simulink model "ExampleMotive_control_communication"  (R2016a)
settings: Solver=ode1  StartTime=0.0  StopTime=inf  FixedStep=0.2  RelTol=1e-3
settings Model: ExtModeTrigDuration=5000  Creator=adm-drone  LastModifiedBy=jitesh_esb201
settings SolverCC: PositivePriorityOrder=on
settings DataIOCC: LimitDataPoints=on  SaveFormat=Array
settings DebuggingCC: UnderspecifiedInitializationDetection=Classic  MergeDetectMultiDrivingBlocksExec=none  SolverPrmCheckMsg=warning  StateNameClashWarn=warning
settings HardwareCC: ProdBitPerPointer=32  ProdLargestAtomicFloat=None  ProdIntDivRoundTo=Undefined  ProdEndianess=Unspecified  ProdWordSize=32  ProdHWDeviceType=32-bit Generic
settings ModelReferenceCC: PropagateSignalLabelsOutOfModel=off
settings RTWCC: SystemTargetFile=quarc_win64.tlc  TemplateMakefile=quarc_default_tmf  Description=QUARC Win64 Target
settings STFCustomTargetCC: TargetPreCompLibLocation=C:\PROGRA~3\QUARC\lib\2013a\win64\release  GeneratePreprocessorConditionals=Disable all  CombineOutputUpdateFcns=on  CPPClassGenCompliant=on  GRTInterface=off  SystemTargetFile=quarc_win64.tlc
settings GRTTargetCC: TargetPreCompLibLocation=C:\PROGRA~3\QUARC\lib\2013a\win64\release  ParMdlRefBuildCompliant=off  CompOptLevelCompliant=off  ConcurrentExecutionCompliant=off  MatFileLogging=off  UseToolchainInfoCompliant=off  ExtMode=on  ExtModeMexFile=quarc_comm
settings ConfigComp: CovModelRefEnable=Off

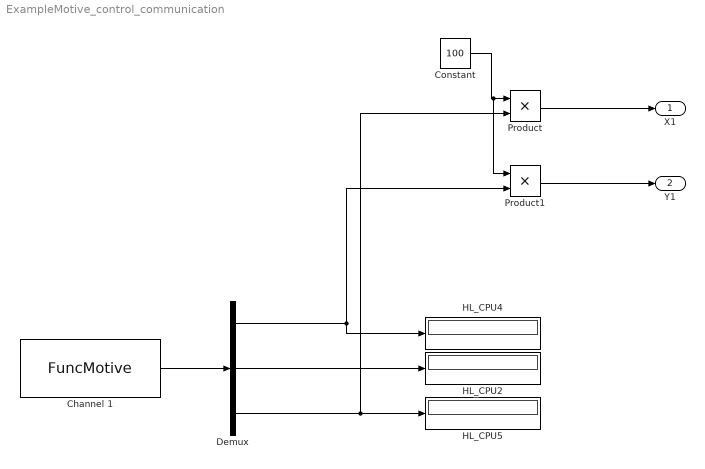
== system ExampleMotive_control_communication ==
  Channel 1 : M-S-Function  FunctionName=FuncMotive  Parameters=1
  Constant : Constant  Value=100
  Demux : Demux  Outputs=3
  HL_CPU2 : Display
  HL_CPU4 : Display
  HL_CPU5 : Display
  Product : Product
  Product1 : Product
  X1 : Outport
  Y1 : Outport  Port=2
  wires:
  Channel 1/1 -> Demux/1
  Demux/1 -> HL_CPU4/1, Product1/2
  Demux/2 -> HL_CPU2/1
  Demux/3 -> Product/2, HL_CPU5/1
  Constant/1 -> Product1/1, Product/1
  Product/1 -> X1/1
  Product1/1 -> Y1/1
